simulink model "finalsimulink"  (R2023b)
settings: Solver=VariableStepAuto  StartTime=1e-10  StopTime=1  RelTol=1e-3
libraries: spsMosfetLib x8, spsSeriesRLCBranchLib x5, spsCurrentMeasurementLib x2, spsDCVoltageSourceLib x2, simulink_extras x2, spsSawtoothGeneratorLib x2, spsVoltageMeasurementLib x2, spsStairGeneratorLib x1, spsMeanLib x1, slpidlib x1, spsOnDelayLib x1, spsVariableRatioTransformerLib x1
settings Model: Creator=abhis  LastModifiedBy=abhis

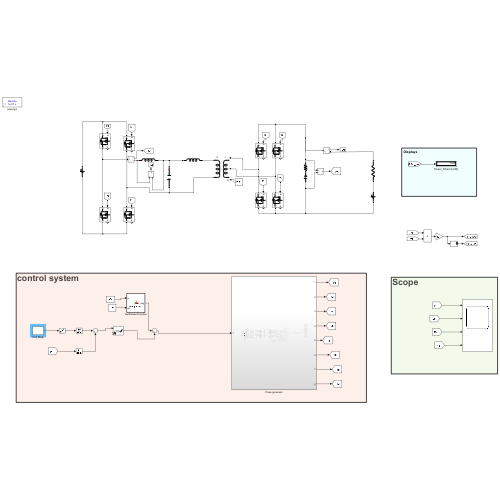
[thumbnail: Simulink's stored preview of the top-level diagram]
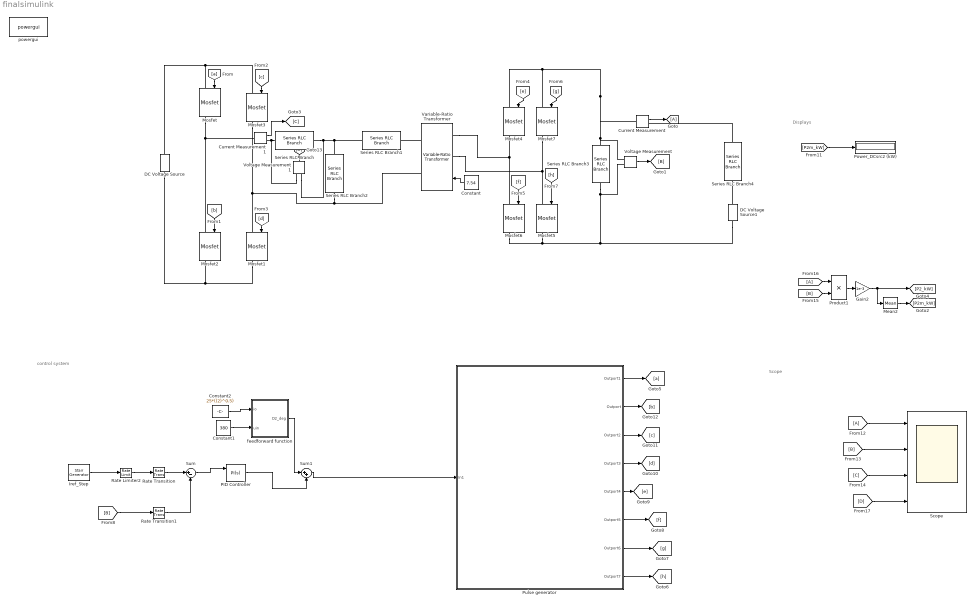
== system finalsimulink ==
  note: Scope
  note: control system
  note: Displays
  Constant : Constant  Value=7.54
  Constant1 : Constant  Value=380
  Constant2 : Constant  Value=25*((2)^0.5)
  Current Measurement : spsCurrentMeasurementLib/Current Measurement  PhasorSimulation=off  OutputType=Complex  PSBequivalent=0
  Current Measurement1 : spsCurrentMeasurementLib/Current Measurement  PhasorSimulation=off  OutputType=Complex  PSBequivalent=0
  DC Voltage Source : spsDCVoltageSourceLib/DC Voltage Source  Amplitude=380  Measurements=None
  DC Voltage Source1 : spsDCVoltageSourceLib/DC Voltage Source  Amplitude=55  Measurements=None
  From12 : From
  From16 : From
  Gain2 : Gain  Gain=1e-3
  Goto : Goto
  Iref_Step : spsStairGeneratorLib/Stair Generator  t=[1e-10, 0.01]  e=[100, -0.001]  Ts=0
  Mean2 : spsMeanLib/Mean  Freq=50  Vinit=0  Ts=0
  Mosfet{,1..7} (8 alike) : spsMosfetLib/Mosfet  Ron=0.1  Lon=0  Rd=0.01  Vfd=0  IC=0  Rs=1e5  Cs=inf  Measurements=on
  PID Controller : slpidlib/PID Controller  Controller=PI  Form=Parallel  TimeDomain=Continuous-time  UseExternalTs=off  SampleTime=-1  IntegratorMethod=Forward Euler  FilterMethod=Forward Euler  ControllerParametersSource=internal  P=0.1  I=5000  UseKiTs=on  D=0  N=100  UseFilter=on  TunerSelectOption=Transfer Function Based (PID Tuner App)  InitialConditionSource=internal  InitialConditionForIntegrator=0  InitialConditionForFilter=0  DifferentiatorICPrevScaledInput=0  ExternalReset=falling  TrackingMode=off  Kt=1  LimitOutput=on  SatLimitsSource=internal  UpperSaturationLimit=50  LowerSaturationLimit=-50  LinearizeAsGain=on  AntiWindupMode=clamping  Kb=1  LimitIntegrator=off  UpperIntegratorSaturationLimit=inf  LowerIntegratorSaturationLimit=-inf  PGainOutDataTypeStr=Inherit: Keep MSB  PProdOutDataTypeStr=Inherit: Keep MSB  POutMin=[]  POutMax=[]  IOutMin=[]  IOutMax=[]  DOutMin=[]  DOutMax=[]  NOutMin=[]  NOutMax=[]  SumOutMin=[]  SumOutMax=[]  SaturationOutMin=[]  SaturationOutMax=[]  PParamMin=[]  PParamMax=[]  IParamMin=[]  IParamMax=[]  DParamMin=[]  DParamMax=[]  NParamMin=[]  NParamMax=[]  KbParamMin=[]  KbParamMax=[]  KtParamMin=[]  KtParamMax=[]  KbOutMin=[]  KbOutMax=[]  KtOutMin=[]  KtOutMax=[]  IntegratorOutMin=[]  IntegratorOutMax=[]  FilterOutMin=[]  FilterOutMax=[]  SumI1OutMin=[]  SumI1OutMax=[]  SumI2OutMin=[]  SumI2OutMax=[]  SumI3OutMin=[]  SumI3OutMax=[]  SumI4OutMin=[]  SumI4OutMax=[]  SumDOutMin=[]  SumDOutMax=[]  DifferentiatorOutMin=[]  DifferentiatorOutMax=[]  FilterDiffOutCoefMin=[]  FilterDiffOutCoefMax=[]  ReciprocalOutMin=[]  ReciprocalOutMax=[]  SumDenOutMin=[]  SumDenOutMax=[]  SumNumOutMin=[]  SumNumOutMax=[]  DivideOutMin=[]  DivideOutMax=[]  UdiffTsProdOutMin=[]  UdiffTsProdOutMax=[]  NTsProdOutMin=[]  NTsProdOutMax=[]  UintegralTsProdOutMin=[]  UintegralTsProdOutMax=[]  UngainTsProdOutMin=[]  UngainTsProdOutMax=[]  ClampingZeroOutDataTypeStr=Inherit: Inherit via back propagation  ClampingZeroOutMin=[]  ClampingZeroOutMax=[]  FilterDenConstantOutDataTypeStr=Inherit: Inherit via back propagation  FilterDenConstantOutMin=[]  FilterDenConstantOutMax=[]  PCopyOutDataTypeStr=Inherit: Inherit via back propagation  PCopyOutMin=[]  PCopyOutMax=[]  NCopyOutDataTypeStr=Inherit: Inherit via back propagation  NCopyOutMin=[]  NCopyOutMax=[]  IntegratorContinuousStateAttributes=''  IntegratorStateMustResolveToSignalObject=off  IntegratorRTWStateStorageClass=Auto  FilterContinuousStateAttributes=''  FilterStateMustResolveToSignalObject=off  FilterRTWStateStorageClass=Auto  ParallelPVariant=InternalParameters  IdealPVariant=Disabled  IVariant=InternalParameters  DVariant=Disabled  IntegratorVariant=Continuous  SatVariant=Enabled  AWVariant=ContClampingParallel  PCopyVariant=Disabled  TRVariant=Disabled  FdbkBlocksVariant=Forward  IdealPFdbkVariant=Disabled  SatFdbkVariant=Disabled  DerivativeFilterVariant=Disabled  NVariant=Disabled  NCopyVariant=Disabled_SignalSpec  FilterICVariant=Disabled  IntegratorICVariant=InternalICs  ExternalResetVariant=ExternalReset  TRSumVariant=Passthrough  SumFdbkVariant=Disabled  SumVariant=Sum_PI  TsampFilterVariant=InternalTs  TsampNgainVariant=Passthrough  TsampIntegralVariant=Disabled_SignalSpec  ExternalSaturationOutDataTypeStr=Inherit: Same as second input
  Power_DCsrc2 (kW) : Display
      settings: Format=bank  Decimation=100
  Product1 : Product
  Pulse generator : Subsystem
  Rate Limiter2 : RateLimiter  RisingSlewLimit=3000  FallingSlewLimit=-3000  SampleTimeMode=inherited
  Rate Transition : RateTransition  OutPortSampleTimeOpt=Inherit  OutPortSampleTime=Ts_Control
  Rate Transition1 : RateTransition  OutPortSampleTimeOpt=Inherit  OutPortSampleTime=Ts_Control
  Scope : Scope  NumInputPorts=4
  Series RLC Branch : spsSeriesRLCBranchLib/Series RLC Branch  LConnTagsString=__new0  RConnTagsString=__new0  BranchType=L  Resistance=1  Inductance=145e-06  SetiL0=off  InitialCurrent=0  Capacitance=1e-6  Setx0=off  InitialVoltage=0  Measurements=None
  Series RLC Branch1 : spsSeriesRLCBranchLib/Series RLC Branch  LConnTagsString=__new0  RConnTagsString=__new0  BranchType=L  Resistance=1  Inductance=145e-06  SetiL0=off  InitialCurrent=0  Capacitance=1e-6  Setx0=off  InitialVoltage=0  Measurements=None
  Series RLC Branch2 : spsSeriesRLCBranchLib/Series RLC Branch  LConnTagsString=__new0  RConnTagsString=__new0  BranchType=C  Resistance=1  Inductance=1e-3  SetiL0=off  InitialCurrent=0  Capacitance=7e-08  Setx0=off  InitialVoltage=0  Measurements=None
  Series RLC Branch3 : spsSeriesRLCBranchLib/Series RLC Branch  LConnTagsString=__new0  RConnTagsString=__new0  BranchType=RC  Resistance=10  Inductance=1e-3  SetiL0=off  InitialCurrent=0  Capacitance=5e-4  Setx0=off  InitialVoltage=0  Measurements=None
  Series RLC Branch4 : spsSeriesRLCBranchLib/Series RLC Branch  LConnTagsString=__new0  RConnTagsString=__new0  BranchType=R  Resistance=10  Inductance=1e-3  SetiL0=off  InitialCurrent=0  Capacitance=1e-6  Setx0=off  InitialVoltage=0  Measurements=None
  Sum : Sum  Inputs=|+-
  Sum1 : Sum  Inputs=|++
  Variable-Ratio Transformer : spsVariableRatioTransformerLib/Variable-Ratio Transformer
      settings: LibrarySourceBlock=|
      | sps_lib/Passives/Variable-Ratio
      | Transformer
  Voltage Measurement : spsVoltageMeasurementLib/Voltage Measurement  PhasorSimulation=off  OutputType=Complex  PSBequivalent=0
  Voltage Measurement1 : spsVoltageMeasurementLib/Voltage Measurement  PhasorSimulation=off  OutputType=Complex  PSBequivalent=0
  feedforward function : MATLAB Function  TreatAsAtomicUnit=on
  powergui : sps_lib/powergui  Priority=1  SimulationMode=Discrete  SampleTime=1e-07  frequency=60  Iterations=50  frequencyindice=0  Pbase=100e6  ErrMax=1e-4  UnitsV=kV  UnitsW=MW  buscounter=0  FunctionMessages=off  echomessages=off  EnableUseOfTLC=off  CurrentSourceSwitches=off  DisableSnubberDevices=off  DisableRonSwitches=off  DisableVfSwitches=off  DisplayEquations=off  AutomaticDiscreteSolvers=off  SolverType=Tustin/Backward Euler (TBE)  Interpol=off  ExternalGateDelay=off  methode=off  Ts=100  x0status=blocks  SPID=on  SwTol=0  HookPort=off  NonlinearTolerance=1e-4  nMaxIteration=100  ContinueOnMaxIteration=off  RestoreLinks=warning  ResistiveCurrentMeasurement=off  Frange=[0:2:500]  Ylog=off  Xlog=on  ShowGrid=off  save=off  variable=ZData  structure=0  ZoomFFT=off  StartTime=0.0  cycles=1  DisplayStyle=1  fundamental=60  FreqAxis=off  MaxFrequency=1000  frequencyindicesteady=1  RmsSteady=1  display=off
  wires:
  Constant/1 -> Variable-Ratio Transformer/1
  [a] -> Mosfet/1
  [b] -> Mosfet2/1
  [c] -> Mosfet3/1
  [d] -> Mosfet1/1
  [e] -> Mosfet4/1
  [f] -> Mosfet6/1
  [g] -> Mosfet7/1
  [h] -> Mosfet5/1
  Current Measurement/1 -> Goto/1
  Voltage Measurement/1 -> [B]
  [B] -> Rate Transition1/1
  feedforward function/1(D2_deg) -> Sum1/1
  Gain2/1 -> Mean2/1, [P2_kW]
  Mean2/1 -> [P2m_kW]
  Product1/1 -> Gain2/1
  From16/1 -> Product1/1
  [B] -> Product1/2
  [P2m_kW] -> Power_DCsrc2 (kW)/1
  Current Measurement1/1 -> [C]
  From12/1 -> Scope/1
  [B] -> Scope/2
  [C] -> Scope/3
  [D] -> Scope/4
  Pulse generator/1(Outport1) -> [a]
  Pulse generator/2(Outport) -> [b]
  Pulse generator/3(Outport2) -> [c]
  Pulse generator/4(Outport3) -> [d]
  Pulse generator/5(Outport4) -> [e]
  Pulse generator/6(Outport5) -> [f]
  Pulse generator/7(Outport6) -> [g]
  Pulse generator/8(Outport7) -> [h]
  PID Controller/1 -> Sum1/2
  Sum/1 -> PID Controller/1
  Sum1/1 -> Pulse generator/1(In1)
  Voltage Measurement1/1 -> [D]
  Iref_Step/1 -> Rate Limiter2/1
  Rate Limiter2/1 -> Rate Transition/1
  Rate Transition/1 -> Sum/1
  Rate Transition1/1 -> Sum/2
  Constant1/1 -> feedforward function/2(uin)
  Constant2/1 -> feedforward function/1(io)
  connections:
  DC Voltage Source/RConn1 -- Mosfet3/LConn1 -- Mosfet/LConn1
  DC Voltage Source/LConn1 -- Mosfet2/RConn1 -- Mosfet1/RConn1
  Mosfet/RConn1 -- Current Measurement1/LConn1 -- Mosfet2/LConn1
  Mosfet3/RConn1 -- Variable-Ratio Transformer/RConn1 -- Series RLC Branch2/RConn1 -- Mosfet1/LConn1
  Series RLC Branch/RConn1 -- Series RLC Branch1/LConn1 -- Series RLC Branch2/LConn1 -- Voltage Measurement1/LConn2
  Variable-Ratio Transformer/RConn2 -- Series RLC Branch1/RConn1
  Mosfet4/LConn1 -- Mosfet7/LConn1 -- Voltage Measurement/LConn1 -- Series RLC Branch3/LConn1 -- Current Measurement/LConn1
  Mosfet6/RConn1 -- Voltage Measurement/LConn2 -- Series RLC Branch3/RConn1 -- DC Voltage Source1/LConn1 -- Mosfet5/RConn1
  Mosfet7/RConn1 -- Variable-Ratio Transformer/LConn1 -- Mosfet5/LConn1
  Mosfet6/LConn1 -- Variable-Ratio Transformer/LConn2 -- Mosfet4/RConn1
  Current Measurement1/RConn1 -- Series RLC Branch/LConn1 -- Voltage Measurement1/LConn1
  DC Voltage Source1/RConn1 -- Series RLC Branch4/RConn1
  Series RLC Branch4/LConn1 -- Current Measurement/RConn1

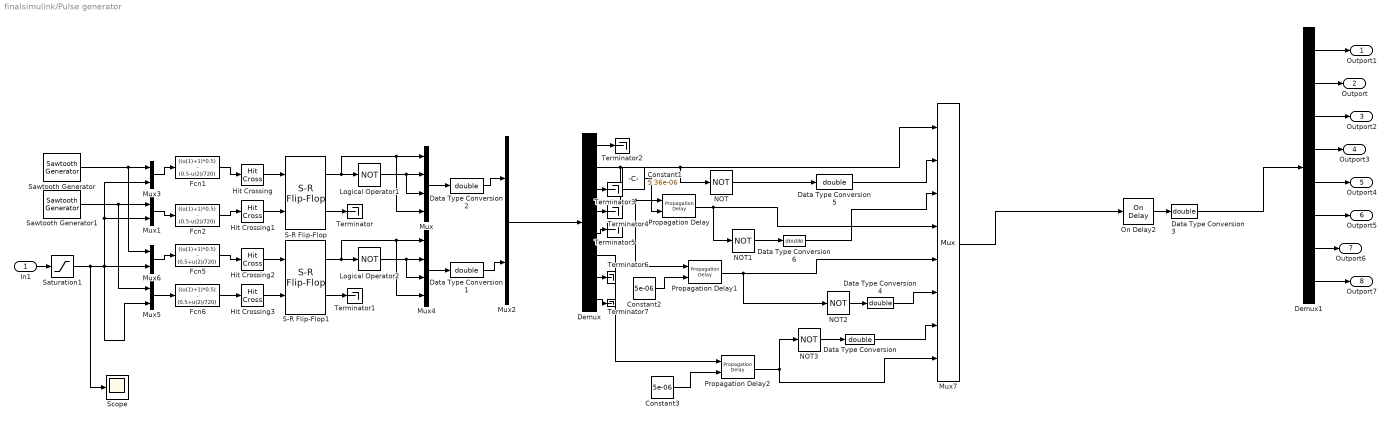
== system finalsimulink/Pulse generator ==
  In1 : Inport
  Constant1 : Constant  Value=5.36e-06
  Constant2 : Constant  Value=5e-06
  Constant3 : Constant  Value=5e-06
  Data Type Conversion{,1..6} (7 alike) : DataTypeConversion  OutDataTypeStr=double  SaturateOnIntegerOverflow=off  RndMeth=Floor
  Demux : Demux  Outputs=8
  Demux1 : Demux  Outputs=8
  Fcn1 : Fcn  Expr=((u(1)+1)*0.5) - (0.5-u(2)/720)
  Fcn2 : Fcn  Expr=((u(1)+1)*0.5) - (0.5-u(2)/720)
  Fcn5 : Fcn  Expr=((u(1)+1)*0.5) - (0.5+u(2)/720)
  Fcn6 : Fcn  Expr=((u(1)+1)*0.5) - (0.5+u(2)/720)
  Hit Crossing{,1..3} (4 alike) : HitCross  HitCrossingDirection=rising
  Logical Operator1 : Logic  Operator=NOT  AllPortsSameDT=off  OutDataTypeStr=boolean
  Logical Operator2 : Logic  Operator=NOT  AllPortsSameDT=off  OutDataTypeStr=boolean
  Mux : Mux
  Mux{1,3,5..6} (4 alike) : Mux  Inputs=2
  Mux2 : Mux  Inputs=[4,4]
  Mux4 : Mux
  Mux7 : Mux  Inputs=8
  NOT{,1..3} (4 alike) : Logic  Operator=NOT  AllPortsSameDT=off  OutDataTypeStr=boolean
  On Delay2 : spsOnDelayLib/On Delay  DelayType=On delay  delay=5e-08  ic=0  Ts=0
  Propagation Delay : PropagationDelay
  Propagation Delay1 : PropagationDelay
  Propagation Delay2 : PropagationDelay
  S-R Flip-Flop : simulink_extras/Flip Flops/S-R Flip-Flop  initial_condition=0
  S-R Flip-Flop1 : simulink_extras/Flip Flops/S-R Flip-Flop  initial_condition=0
  Saturation1 : Saturate  UpperLimit=300  LowerLimit=-300
  Sawtooth Generator : spsSawtoothGeneratorLib/Sawtooth Generator  Freq=50000  Phase=0  Ts=0
  Sawtooth Generator1 : spsSawtoothGeneratorLib/Sawtooth Generator  Freq=50000  Phase=180  Ts=0
  Scope : Scope
  Terminator{,1..7} (8 alike) : Terminator
  Outport1 : Outport
  Outport : Outport  Port=2
  Outport2 : Outport  Port=3
  Outport3 : Outport  Port=4
  Outport4 : Outport  Port=5
  Outport5 : Outport  Port=6
  Outport6 : Outport  Port=7
  Outport7 : Outport  Port=8
  wires:
  Hit Crossing3/1 -> S-R Flip-Flop1/2
  Sawtooth Generator/1 -> Mux6/1, Mux3/1
  Demux/2 -> NOT/1, Mux7/1, Propagation Delay1/1, Propagation Delay/1
  S-R Flip-Flop/1 -> Mux/4, Mux/1, Logical Operator1/1
  Hit Crossing/1 -> S-R Flip-Flop/1
  Mux1/1 -> Fcn2/1
  Propagation Delay2/1 -> Mux7/8, NOT3/1
  Sawtooth Generator1/1 -> Mux5/1, Mux1/1
  Data Type Conversion1/1 -> Mux2/2
  Hit Crossing1/1 -> S-R Flip-Flop/2
  Constant2/1 -> Propagation Delay1/2
  NOT3/1 -> Data Type Conversion/1
  Constant3/1 -> Propagation Delay2/2
  Logical Operator2/1 -> Mux4/3, Mux4/2
  Mux7/1 -> On Delay2/1
  Propagation Delay/1 -> NOT1/1, Mux7/4
  NOT2/1 -> Data Type Conversion4/1
  Mux/1 -> Data Type Conversion2/1
  Constant1/1 -> Propagation Delay/2
  Mux6/1 -> Fcn5/1
  Saturation1/1 -> Scope/1, Mux6/2, Mux5/2, Mux1/2, Mux3/2
  Fcn6/1 -> Hit Crossing3/1
  Mux2/1 -> Demux/1
  Logical Operator1/1 -> Mux/2, Mux/3
  Propagation Delay1/1 -> NOT2/1, Mux7/5
  Fcn5/1 -> Hit Crossing2/1
  Hit Crossing2/1 -> S-R Flip-Flop1/1
  S-R Flip-Flop1/1 -> Logical Operator2/1, Mux4/1, Mux4/4
  Data Type Conversion2/1 -> Mux2/1
  NOT1/1 -> Data Type Conversion6/1
  Fcn2/1 -> Hit Crossing1/1
  S-R Flip-Flop/2 -> Terminator/1
  Fcn1/1 -> Hit Crossing/1
  On Delay2/1 -> Data Type Conversion3/1
  Demux/6 -> Propagation Delay2/1
  Data Type Conversion3/1 -> Demux1/1
  Mux3/1 -> Fcn1/1
  NOT/1 -> Data Type Conversion5/1
  Mux4/1 -> Data Type Conversion1/1
  Mux5/1 -> Fcn6/1
  S-R Flip-Flop1/2 -> Terminator1/1
  In1/1 -> Saturation1/1
  Demux/1 -> Terminator2/1
  Demux/3 -> Terminator3/1
  Demux/4 -> Terminator4/1
  Demux/5 -> Terminator5/1
  Demux/7 -> Terminator6/1
  Demux/8 -> Terminator7/1
  Data Type Conversion/1 -> Mux7/7
  Data Type Conversion4/1 -> Mux7/6
  Data Type Conversion5/1 -> Mux7/2
  Data Type Conversion6/1 -> Mux7/3
  Demux1/1 -> Outport1/1
  Demux1/2 -> Outport/1
  Demux1/3 -> Outport2/1
  Demux1/4 -> Outport3/1
  Demux1/5 -> Outport4/1
  Demux1/6 -> Outport5/1
  Demux1/7 -> Outport6/1
  Demux1/8 -> Outport7/1

== matlab function finalsimulink/feedforward function ==
  data: io input; D2_deg output; uin input
function D2_deg = computeD2(io, uin)
%#codegen
% Computes the phase angle D2 in degrees based on io and uin inputs

% Define kff as pi^2 / 16
kff = (pi^2) / 16;

% Calculate the argument for acos
x = (kff * io) / uin;

% Clamp x to the valid domain of acos [-1, 1]
x = min(max(x, -1), 1);

% Compute D2 in radians
D2_rad = (1 / pi) * acos(x);

% Convert D2 to degrees
D2_deg = D2_rad * (180 / pi);
end
